simulink model "aero_guidance_targetwith315"  (R2026a)
settings: Solver=FixedStepAuto  StopTime=20  FixedStep=0.001  AbsTol=1e-6
PreLoadFcn:
  | aero_guid_dat
StopFcn:
  | aero_guid_plot
values from neighbouring files (symbols this model uses):
  d2r = pi/180    (= 0.0174532925199)    [aero_guid_plot.m]
  target_dt = 0.01    [rl_target_params.m]
undefined symbols (not defined in the file or in its folder): alpha_sch, alpha_vec, Beamwidth, Cm_alpha, Cm_el, Cm_q, Cx_alpha, Cz_alpha, Cz_el, d_ref, fin_max, fin_min, g, h_ini, K, K_r, Ka, Kg, Ki, Ks, l_acc, M_sch, Mach_vec, max_acc, max_gimbal, min_gimbal, omegaDotMax, omegaPhysMax, pos_tgt, q_ini, S_ref, Thrust, tors, v_ini, v_tgt, wgyro, wn_hom, x_ini
libraries: aerolibasang x3, simulink x2, aerolibanim x1, aerolibatmos2 x1, aerolibactuator x1, rllib x1
(part 1 of 2)
CloseFcn:
  | h=findobj('type','figure');if ~isempty(h);close(h);end
Description:
  | Dynamics of a missile engaging a target which is flying straight and level
settings Model: ExtModeTrigMode=oneshot  ExtModeArmWhenConnect=off  ExtModeAutoUpdateStatusClock=off  Creator=The MathWorks, Inc.  LastModifiedBy=신예현
settings DataIOCC: StateSaveName=xbase  OutputSaveName=ybase  SignalLoggingName=sigsOut
settings OptimizationCC: InitFltsAndDblsToZero=on
settings DebuggingCC: SaveWithParameterizedLinksMsg=none  SignalResolutionControl=TryResolveAllWithWarning  MultiTaskDSMMsg=warning  MultiTaskCondExecSysMsg=none  SigSpecEnsureSampleTimeMsg=none
settings HardwareCC: ProdHWDeviceType=32-bit Generic
settings GRTTargetCC: TargetFcnLib=ansi_tfl_tmw.mat  CombineOutputUpdateFcns=off  GRTInterface=on
settings ConfigComp: CovMetricSettings=d

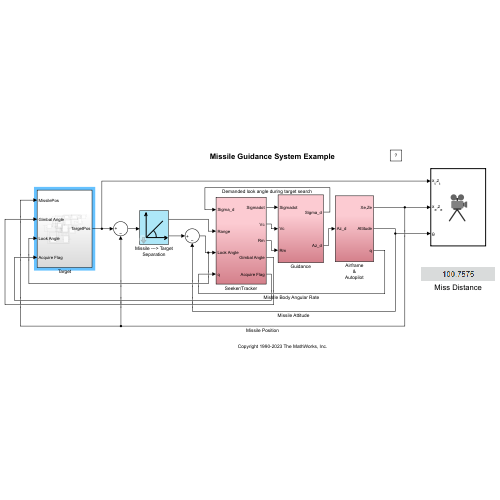
[thumbnail: Simulink's stored preview of the top-level diagram]
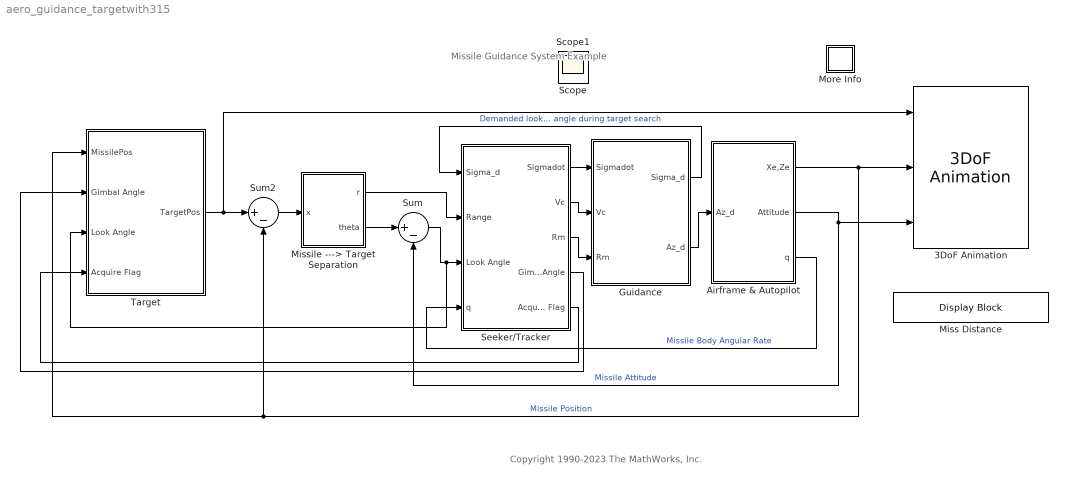
== system aero_guidance_targetwith315 ==
  note: Copyright 1990-2023 The MathWorks, Inc.
  note: Missile Guidance System Example
  3DoF Animation : aerolibanim/3DoF Animation  u1=[0 5000 -2000 2000 -5050 -3500]  u2=0.01  u3=2.0  u5=Fixed position  u6=[2500 8000 -4000]  u7=35  u8=on
  Airframe & Autopilot : Subsystem
  Guidance : Subsystem
  Miss Distance : DisplayBlock  LabelPosition=Hide  Transparency=1  GridColor=[0.0, 0.0, 0.0]
  Missile ---> Target Separation : Subsystem  mask(Cart2Polar){}
      mask help:
      | Transformation from cartesian to polar coordinates.
      | [x, y] -> [r, theta]
      |
      | r = sqrt(x^2 + y^2);
      | theta = atan(y/x);
      mask Help: Unmask this block for more help.
      mask Display: plot(0,0,100,100,[24,20,15,20,20],[85,95,85,95,20],[80,20,95,85,95,85],[70,20,20,15,20,24],[56,56,55,52,50,46],[20,26,31,35,38,42])
  More Info : Subsystem
      settings: OpenFcn=showExample('simulink_aerospace/DesigningAGuidanceSystemInMATLABAndSimulinkExample')
      mask Display: disp('?')
  Seeker/Tracker : Subsystem
  Sum : Sum  Inputs=|+-  InputSameDT=on  SaturateOnIntegerOverflow=on  OutDataTypeStr=Inherit: Same as first input
  Sum2 : Sum  Inputs=|+-  InputSameDT=on  SaturateOnIntegerOverflow=on  OutDataTypeStr=Inherit: Same as first input
  Target : Subsystem
  Scope : Scope
  Scope1 : Scope
  wires:
  Missile ---> Target Separation/2(theta) -> Sum/1
  Guidance/2(Az_d) -> Airframe & Autopilot/1(Az_d)
  Seeker/Tracker/2(Vc) -> Guidance/2(Vc)
  Seeker/Tracker/3(Rm) -> Guidance/3(Rm)
  Seeker/Tracker/1(Sigmadot) -> Guidance/1(Sigmadot)
  Sum/1 -> Target/3(Look Angle), Seeker/Tracker/3(Look Angle)
  Airframe & Autopilot/3(q) -> Seeker/Tracker/4(q)  "Missile Body Angular Rate"
  Guidance/1(Sigma_d) -> Seeker/Tracker/1(Sigma_d)  "Demanded look angle during target search"
  Missile ---> Target Separation/1(r) -> Seeker/Tracker/2(Range)
  Airframe & Autopilot/1(Xe,Ze) -> Target/1(MissilePos), Sum2/2, 3DoF Animation/2  "Missile Position"
  Airframe & Autopilot/2(Attitude) -> Sum/2, 3DoF Animation/3  "Missile Attitude"
  Sum2/1 -> Missile ---> Target Separation/1(x)
  Target/1(TargetPos) -> 3DoF Animation/1, Sum2/1
  Seeker/Tracker/4(Gimbal Angle) -> Target/2(Gimbal Angle)
  Seeker/Tracker/5(Acquire Flag) -> Target/4(Acquire Flag)

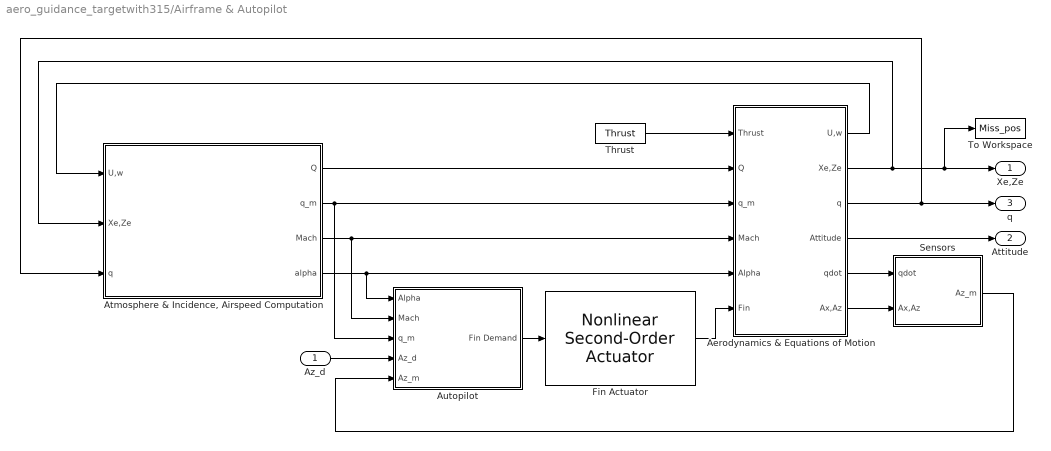
== system aero_guidance_targetwith315/Airframe & Autopilot ==
  Az_d : Inport
  Aerodynamics & Equations of Motion : Subsystem
  "Atmosphere & Incidence, Airspeed Computation" : Subsystem
  Autopilot : Subsystem
  Fin Actuator : aerolibactuator/Nonlinear Second-Order Actuator  wn_fin=wn_fin  z_fin=z_fin  fin_max=fin_max  fin_min=fin_min  fin_maxrate=fin_maxrate  fin_act_0=fin_act_0  fin_act_vel=0
  Sensors : Subsystem
  Thrust : Constant  Value=Thrust
  To Workspace : ToWorkspace  VariableName=Miss_pos  SaveFormat=Structure With Time  SampleTime=-1
  Xe,Ze : Outport  InitialOutput=0  VectorParamsAs1DForOutWhenUnconnected=off
  Attitude : Outport  Port=2  InitialOutput=0  VectorParamsAs1DForOutWhenUnconnected=off
  q : Outport  Port=3  InitialOutput=0  VectorParamsAs1DForOutWhenUnconnected=off
  wires:
  Thrust/1 -> Aerodynamics & Equations of Motion/1(Thrust)
  Aerodynamics & Equations of Motion/3(q) -> q/1, "Atmosphere & Incidence, Airspeed Computation"/3(q)
  Aerodynamics & Equations of Motion/2(Xe,Ze) -> To Workspace/1, Xe,Ze/1, "Atmosphere & Incidence, Airspeed Computation"/2(Xe,Ze)
  "Atmosphere & Incidence, Airspeed Computation"/3(Mach) -> Aerodynamics & Equations of Motion/4(Mach), Autopilot/2(Mach)
  Aerodynamics & Equations of Motion/1(U,w) -> "Atmosphere & Incidence, Airspeed Computation"/1(U,w)
  "Atmosphere & Incidence, Airspeed Computation"/1(Q) -> Aerodynamics & Equations of Motion/2(Q)
  "Atmosphere & Incidence, Airspeed Computation"/4(alpha) -> Autopilot/1(Alpha), Aerodynamics & Equations of Motion/5(Alpha)
  "Atmosphere & Incidence, Airspeed Computation"/2(q_m) -> Aerodynamics & Equations of Motion/3(q_m), Autopilot/3(q_m)
  Aerodynamics & Equations of Motion/4(Attitude) -> Attitude/1
  Aerodynamics & Equations of Motion/5(qdot) -> Sensors/1(qdot)
  Aerodynamics & Equations of Motion/6(Ax,Az) -> Sensors/2(Ax,Az)
  Autopilot/1(Fin Demand) -> Fin Actuator/1
  Fin Actuator/1 -> Aerodynamics & Equations of Motion/6(Fin)
  Az_d/1 -> Autopilot/4(Az_d)
  Sensors/1(Az_m) -> Autopilot/5(Az_m)

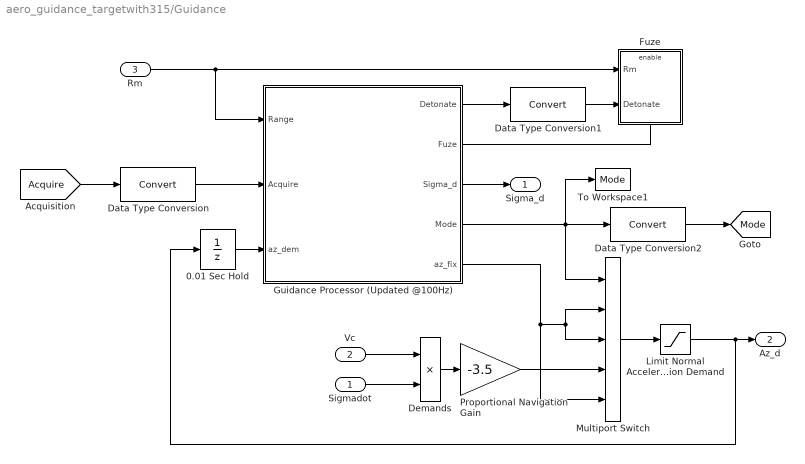
== system aero_guidance_targetwith315/Guidance ==
  Sigmadot : Inport
  Vc : Inport  Port=2
  Rm : Inport  Port=3
  0.01 Sec Hold : UnitDelay  SampleTime=0.01
  Data Type Conversion : DataTypeConversion  SaturateOnIntegerOverflow=off  RndMeth=Floor
  Data Type Conversion1 : DataTypeConversion  SaturateOnIntegerOverflow=off  RndMeth=Floor
  Data Type Conversion2 : DataTypeConversion  SaturateOnIntegerOverflow=off  RndMeth=Floor
  Demands : Product  InputSameDT=on  SaturateOnIntegerOverflow=on  OutDataTypeStr=Inherit: Same as first input
  Fuze : Subsystem  TreatAsAtomicUnit=on
  Guidance Processor (Updated @100Hz) : Stateflow chart  TreatAsAtomicUnit=on
  "Limit Normal Acceleration Demand " : Saturate  UpperLimit=max_acc  LowerLimit=-max_acc
  Multiport Switch : MultiPortSwitch  Inputs=4
  Proportional Navigation Gain : Gain  Gain=-3.5  SaturateOnIntegerOverflow=on  OutDataTypeStr=Inherit: Same as input  ParamDataTypeStr=Inherit: Same as input
  To Workspace1 : ToWorkspace  VariableName=Mode  SaveFormat=Structure With Time
  Sigma_d : Outport  VectorParamsAs1DForOutWhenUnconnected=off
  Az_d : Outport  Port=2  VectorParamsAs1DForOutWhenUnconnected=off
  tag scope: Mode=global
  wires:
  Guidance Processor (Updated @100Hz)/3(Sigma_d) -> Sigma_d/1
  [Acquire] -> Data Type Conversion/1
  Multiport Switch/1 -> "Limit Normal Acceleration Demand "/1
  Guidance Processor (Updated @100Hz)/1(Detonate) -> Data Type Conversion1/1
  "Limit Normal Acceleration Demand "/1 -> Az_d/1, 0.01 Sec Hold/1
  Guidance Processor (Updated @100Hz)/5(az_fix) -> Multiport Switch/2, Multiport Switch/3, Multiport Switch/5
  0.01 Sec Hold/1 -> Guidance Processor (Updated @100Hz)/3(az_dem)
  Sigmadot/1 -> Demands/2
  Proportional Navigation Gain/1 -> Multiport Switch/4
  Vc/1 -> Demands/1
  Demands/1 -> Proportional Navigation Gain/1
  Rm/1 -> Fuze/1(Rm), Guidance Processor (Updated @100Hz)/1(Range)
  Guidance Processor (Updated @100Hz)/2(Fuze) -> Fuze/Enable
  Guidance Processor (Updated @100Hz)/4(Mode) -> Data Type Conversion2/1, To Workspace1/1, Multiport Switch/1
  Data Type Conversion/1 -> Guidance Processor (Updated @100Hz)/2(Acquire)
  Data Type Conversion1/1 -> Fuze/2(Detonate)
  Data Type Conversion2/1 -> [Mode]

== system aero_guidance_targetwith315/Missile ---> Target Separation ==
  x : Inport
  Range : Fcn  Expr=hypot(u[1],u[2])
  Sightline Angle : Fcn  Expr=atan2(-u[2],u[1])
  r : Outport  InitialOutput=0  VectorParamsAs1DForOutWhenUnconnected=off
  theta : Outport  Port=2  InitialOutput=0  VectorParamsAs1DForOutWhenUnconnected=off
  wires:
  x/1 -> Sightline Angle/1, Range/1
  Range/1 -> r/1
  Sightline Angle/1 -> theta/1

== system aero_guidance_targetwith315/More Info ==

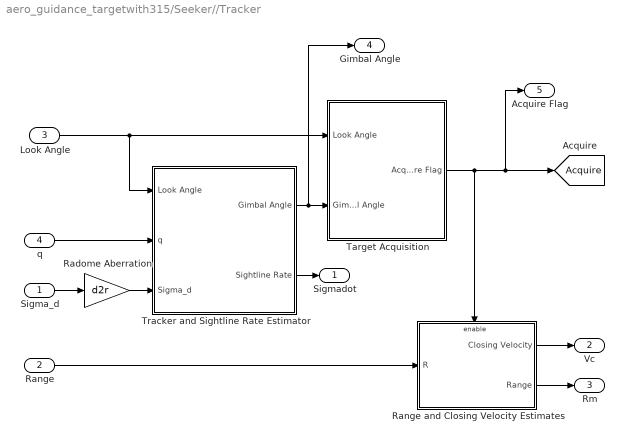
== system aero_guidance_targetwith315/Seeker//Tracker ==
  Sigma_d : Inport
  Range : Inport  Port=2
  Look Angle : Inport  Port=3
  q : Inport  Port=4
  Radome Aberration : Gain  Gain=d2r  SaturateOnIntegerOverflow=on  OutDataTypeStr=Inherit: Same as input  ParamDataTypeStr=Inherit: Same as input
  Range and Closing Velocity Estimates : Subsystem  TreatAsAtomicUnit=on
  Target Acquisition : Subsystem
  Tracker and Sightline Rate Estimator : Subsystem
  Sigmadot : Outport  VectorParamsAs1DForOutWhenUnconnected=off
  Vc : Outport  Port=2  VectorParamsAs1DForOutWhenUnconnected=off
  Rm : Outport  Port=3  VectorParamsAs1DForOutWhenUnconnected=off
  Gimbal Angle : Outport  Port=4
  Acquire Flag : Outport  Port=5
  tag scope: Acquire=global
  wires:
  Tracker and Sightline Rate Estimator/2(Sightline Rate) -> Sigmadot/1
  Radome Aberration/1 -> Tracker and Sightline Rate Estimator/3(Sigma_d)
  Tracker and Sightline Rate Estimator/1("Gimbal Angle ") -> Target Acquisition/2(Gimbal Angle), Gimbal Angle/1
  Target Acquisition/1(Acquire Flag) -> Acquire Flag/1, [Acquire], Range and Closing Velocity Estimates/Enable
  q/1 -> Tracker and Sightline Rate Estimator/2(q)
  Look Angle/1 -> Target Acquisition/1(Look Angle), Tracker and Sightline Rate Estimator/1(Look Angle)
  Range/1 -> Range and Closing Velocity Estimates/1(R)
  Range and Closing Velocity Estimates/2(Range) -> Rm/1
  Range and Closing Velocity Estimates/1(Closing Velocity) -> Vc/1
  Sigma_d/1 -> Radome Aberration/1

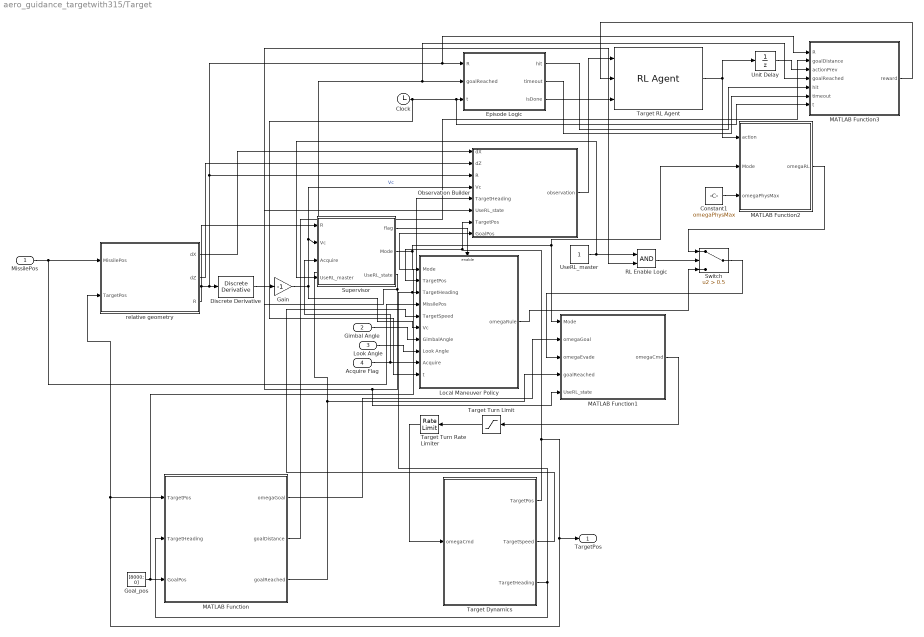
== system aero_guidance_targetwith315/Target ==
  MissilePos : Inport
  Gimbal Angle : Inport  Port=2
  Look Angle : Inport  Port=3
  Acquire Flag : Inport  Port=4
  Clock : Clock
  Constant1 : Constant  Value=omegaPhysMax
  Discrete Derivative : simulink/Discrete/Discrete Derivative  gainval=1.0  ICPrevScaledInput=0.01  OutMin=[]  OutMax=[]  OutDataType=fixdt(1, 16)  OutScaling=2^-10  DoSatur=off
  Episode Logic : MATLAB Function  TreatAsAtomicUnit=on
  Gain : Gain  Gain=-1
  Goal_pos : Constant  Value=[8000; 0]  VectorParams1D=off
  Local Maneuver Policy : Subsystem  TreatAsAtomicUnit=on
  MATLAB Function : MATLAB Function  TreatAsAtomicUnit=on
  MATLAB Function1 : MATLAB Function  TreatAsAtomicUnit=on
  MATLAB Function2 : MATLAB Function  TreatAsAtomicUnit=on
  MATLAB Function3 : MATLAB Function  TreatAsAtomicUnit=on
  Observation Builder : MATLAB Function  TreatAsAtomicUnit=on
  RL Enable Logic : Logic  AllPortsSameDT=off  OutDataTypeStr=boolean
  Supervisor : Stateflow chart  TreatAsAtomicUnit=on
  Switch : Switch  Criteria=u2 > Threshold  Threshold=0.5  SaturateOnIntegerOverflow=off  InputSameDT=off
  Target Dynamics : Subsystem
  Target RL Agent : rllib/RL Agent  Agent=agentObj  ExternalActionAsInput=off  ProvideLastAction=off  ProvideCumRwd=off  TreatAsDirectFeedthrough=on  UseStrictObservationDataTypes=off
  Target Turn Limit : Saturate  UpperLimit=omegaPhysMax  LowerLimit=-omegaPhysMax
  Target Turn Rate Limiter : RateLimiter  RisingSlewLimit=omegaDotMax  FallingSlewLimit=-omegaDotMax  SampleTimeMode=inherited
  Unit Delay : UnitDelay  SampleTime=target_dt
  UseRL_master : Constant
  relative geometry : Subsystem
  TargetPos : Outport
  wires:
  MissilePos/1 -> relative geometry/1(MissilePos), Local Maneuver Policy/4(MissilePos)
  Discrete Derivative/1 -> Gain/1
  relative geometry/3(R) -> Supervisor/1(R), Episode Logic/1(R), MATLAB Function3/1(R), Observation Builder/3(R), Discrete Derivative/1
  Gain/1 -> Observation Builder/4(Vc), Supervisor/2(Vc), Local Maneuver Policy/6(Vc)  "Vc"
  Supervisor/1(flag) -> Local Maneuver Policy/Enable
  Supervisor/2(Mode) -> Local Maneuver Policy/1(Mode), MATLAB Function2/2(Mode), MATLAB Function1/1(Mode)
  Target Dynamics/1(TargetPos) -> Observation Builder/7(TargetPos), Local Maneuver Policy/2(TargetPos), MATLAB Function/1(TargetPos), relative geometry/2(TargetPos), TargetPos/1
  relative geometry/1(dX) -> Observation Builder/1(dX)
  relative geometry/2(dZ) -> Observation Builder/2(dZ)
  Target Dynamics/3(TargetHeading) -> Observation Builder/5(TargetHeading), Local Maneuver Policy/3(TargetHeading), MATLAB Function/2(TargetHeading)
  MATLAB Function/2(goalDistance) -> MATLAB Function3/2(goalDistance)
  MATLAB Function/3(goalReached) -> MATLAB Function3/4(goalReached), Episode Logic/2(goalReached), MATLAB Function1/4(goalReached)
  Goal_pos/1 -> Observation Builder/8(GoalPos), MATLAB Function/3(GoalPos)
  MATLAB Function/1(omegaGoal) -> MATLAB Function1/2(omegaGoal)
  MATLAB Function1/1(omegaCmd) -> Target Turn Limit/1
  Target Turn Limit/1 -> Target Turn Rate Limiter/1
  Target Turn Rate Limiter/1 -> Target Dynamics/1(omegaCmd)
  Local Maneuver Policy/1(omegaRule) -> Switch/3
  Switch/1 -> MATLAB Function1/3(omegaEvade)
  UseRL_master/1 -> Supervisor/4(UseRL_master), RL Enable Logic/1
  Observation Builder/1(observation) -> Target RL Agent/1
  Target RL Agent/1 -> MATLAB Function2/1(action), Unit Delay/1
  MATLAB Function2/1(omegaRL) -> Switch/1
  Clock/1 -> MATLAB Function3/7(t), Episode Logic/3(t), Local Maneuver Policy/10(t)
  Episode Logic/3(isDone) -> Target RL Agent/3
  Unit Delay/1 -> MATLAB Function3/3(actionPrev)
  Episode Logic/1(hit) -> MATLAB Function3/5(hit)
  Episode Logic/2(timeout) -> MATLAB Function3/6(timeout)
  MATLAB Function3/1(reward) -> Target RL Agent/2
  Gimbal Angle/1 -> Local Maneuver Policy/7(GimbalAngle)
  Acquire Flag/1 -> Supervisor/3(Acquire), Local Maneuver Policy/9(Acquire)
  Constant1/1 -> MATLAB Function2/3(omegaPhysMax)
  Look Angle/1 -> Local Maneuver Policy/8(Look Angle)
  Supervisor/3(UseRL_state) -> Observation Builder/6(UseRL_state), MATLAB Function1/5(UseRL_state), RL Enable Logic/2
  RL Enable Logic/1 -> Switch/2
  Target Dynamics/2(TargetSpeed) -> Local Maneuver Policy/5(TargetSpeed)

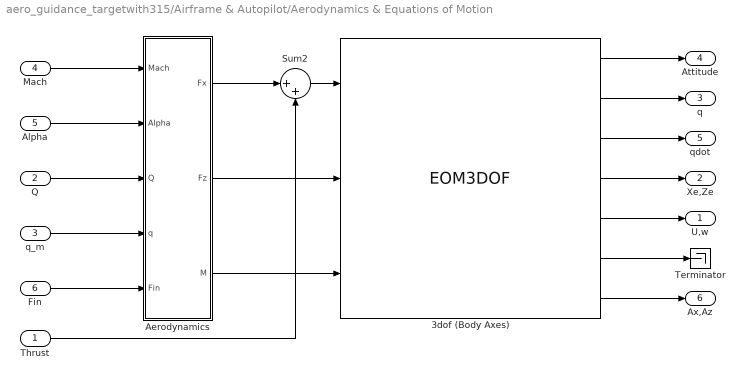
== system aero_guidance_targetwith315/Airframe & Autopilot/Aerodynamics & Equations of Motion ==
  Thrust : Inport
  Q : Inport  Port=2
  q_m : Inport  Port=3
  Mach : Inport  Port=4
  Alpha : Inport  Port=5
  Fin : Inport  Port=6
  3dof (Body Axes) : EOM3DOF  v_ini=v_ini  theta_ini=theta_ini  q_ini=q_ini  alpha_ini=alpha_ini  pos_ini=[x_ini -h_ini]  mass=mass  Iyy=Iyy  g=g  abi_flag=on
  Aerodynamics : Subsystem
  Sum2 : Sum  Inputs=|++  InputSameDT=on  SaturateOnIntegerOverflow=on  OutDataTypeStr=Inherit: Same as first input
  Terminator : Terminator
  U,w : Outport  InitialOutput=0  VectorParamsAs1DForOutWhenUnconnected=off
  Xe,Ze : Outport  Port=2  InitialOutput=0  VectorParamsAs1DForOutWhenUnconnected=off
  q : Outport  Port=3  InitialOutput=0  VectorParamsAs1DForOutWhenUnconnected=off
  Attitude : Outport  Port=4  InitialOutput=0  VectorParamsAs1DForOutWhenUnconnected=off
  qdot : Outport  Port=5  InitialOutput=0  VectorParamsAs1DForOutWhenUnconnected=off
  Ax,Az : Outport  Port=6  InitialOutput=0  VectorParamsAs1DForOutWhenUnconnected=off
  wires:
  Aerodynamics/3(" M") -> 3dof (Body Axes)/3
  Sum2/1 -> 3dof (Body Axes)/1
  Fin/1 -> Aerodynamics/5(Fin)
  Aerodynamics/2(Fz) -> 3dof (Body Axes)/2
  Aerodynamics/1(Fx) -> Sum2/1
  Thrust/1 -> Sum2/2
  q_m/1 -> Aerodynamics/4(q)
  Mach/1 -> Aerodynamics/1(Mach)
  Q/1 -> Aerodynamics/3(Q)
  Alpha/1 -> Aerodynamics/2(Alpha)
  3dof (Body Axes)/7 -> Ax,Az/1
  3dof (Body Axes)/6 -> Terminator/1
  3dof (Body Axes)/5 -> U,w/1
  3dof (Body Axes)/4 -> Xe,Ze/1
  3dof (Body Axes)/3 -> qdot/1
  3dof (Body Axes)/2 -> q/1
  3dof (Body Axes)/1 -> Attitude/1

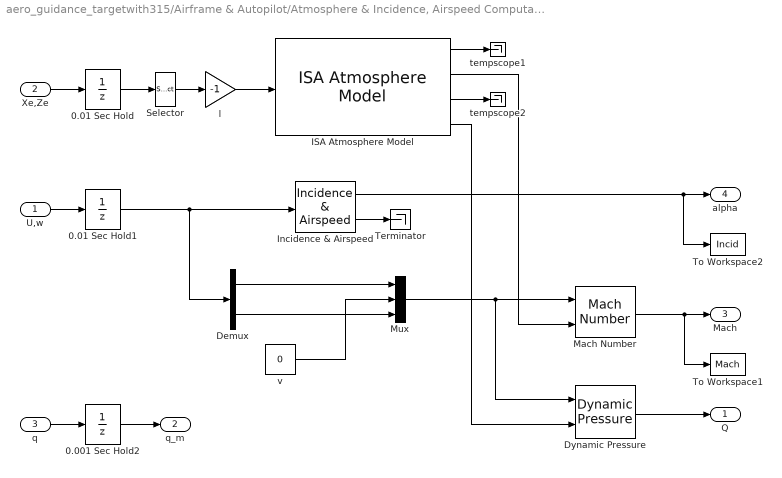
== system aero_guidance_targetwith315/Airframe & Autopilot/Atmosphere & Incidence, Airspeed Computation ==
  U,w : Inport
  Xe,Ze : Inport  Port=2
  q : Inport  Port=3
  0.001 Sec Hold2 : UnitDelay  InitialCondition=q_ini  SampleTime=0.001
  0.01 Sec Hold : UnitDelay  InitialCondition=[x_ini -h_ini]  SampleTime=0.01
  0.01 Sec Hold1 : UnitDelay  InitialCondition=[v_ini 0]  SampleTime=0.01
  Demux : Demux  Outputs=2
  Dynamic Pressure : aerolibasang/Dynamic Pressure
  ISA Atmosphere Model : aerolibatmos2/ISA Atmosphere Model  useExtended=off  action=Warning  custom=off  viscosityOut=off  g=9.80665  gamma=1.4  R=287.0531  L=0.0065  h_trop=11000  h_strat=20000  rho0=1.225  P0=101325  T0=288.15  h0=0  S=110.4  Tref=273.15  muref=1.716e-5
  Incidence & Airspeed : aerolibasang/Incidence  & Airspeed
  Mach Number : aerolibasang/Mach Number
  Mux : Mux  Inputs=3
  Selector : Selector  InputPortWidth=2  IndexOptions=Index vector (dialog)  Indices=[2]  OutputSizes=1
  Terminator : Terminator
  To Workspace1 : ToWorkspace  VariableName=Mach  SaveFormat=Structure With Time  SampleTime=-1
  To Workspace2 : ToWorkspace  VariableName=Incid  SaveFormat=Structure With Time  SampleTime=-1
  l : Gain  Gain=-1  SaturateOnIntegerOverflow=on  OutDataTypeStr=Inherit: Same as input  ParamDataTypeStr=Inherit: Same as input
  tempscope1 : Terminator
  tempscope2 : Terminator
  v : Constant  Value=0
  Q : Outport
  q_m : Outport  Port=2
  Mach : Outport  Port=3
  alpha : Outport  Port=4
  wires:
  U,w/1 -> 0.01 Sec Hold1/1
  Incidence & Airspeed/1 -> To Workspace2/1, alpha/1
  Demux/1 -> Mux/1
  Demux/2 -> Mux/3
  v/1 -> Mux/2
  Mux/1 -> Mach Number/1, Dynamic Pressure/1
  Incidence & Airspeed/2 -> Terminator/1
  ISA Atmosphere Model/4 -> Dynamic Pressure/2
  Mach Number/1 -> To Workspace1/1, Mach/1
  Dynamic Pressure/1 -> Q/1
  0.01 Sec Hold1/1 -> Incidence & Airspeed/1, Demux/1
  0.01 Sec Hold/1 -> Selector/1
  l/1 -> ISA Atmosphere Model/1
  ISA Atmosphere Model/1 -> tempscope1/1
  ISA Atmosphere Model/3 -> tempscope2/1
  Selector/1 -> l/1
  Xe,Ze/1 -> 0.01 Sec Hold/1
  ISA Atmosphere Model/2 -> Mach Number/2
  0.001 Sec Hold2/1 -> q_m/1
  q/1 -> 0.001 Sec Hold2/1

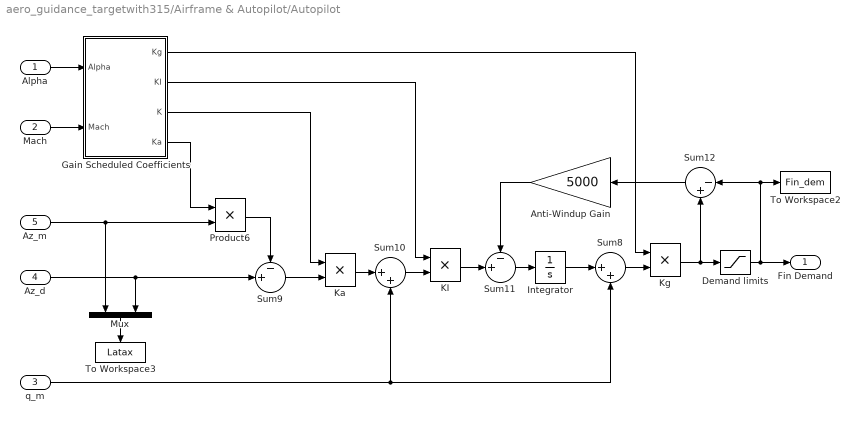
== system aero_guidance_targetwith315/Airframe & Autopilot/Autopilot ==
  Alpha : Inport
  Mach : Inport  Port=2
  q_m : Inport  Port=3
  Az_d : Inport  Port=4
  Az_m : Inport  Port=5
  Anti-Windup Gain : Gain  Gain=5000  SaturateOnIntegerOverflow=on  OutDataTypeStr=Inherit: Same as input  ParamDataTypeStr=Inherit: Same as input
  "Demand limits " : Saturate  UpperLimit=fin_max  LowerLimit=fin_min
  Gain Scheduled Coefficients : Subsystem
  Integrator : Integrator
  KI : Product  InputSameDT=on  SaturateOnIntegerOverflow=on  OutDataTypeStr=Inherit: Same as first input
  Ka : Product  InputSameDT=on  SaturateOnIntegerOverflow=on  OutDataTypeStr=Inherit: Same as first input
  Kg : Product  InputSameDT=on  SaturateOnIntegerOverflow=on  OutDataTypeStr=Inherit: Same as first input
  Mux : Mux  Inputs=2
  Product6 : Product  InputSameDT=on  SaturateOnIntegerOverflow=on  OutDataTypeStr=Inherit: Same as first input
  Sum10 : Sum  Inputs=|++  InputSameDT=on  SaturateOnIntegerOverflow=on  OutDataTypeStr=Inherit: Same as first input
  Sum11 : Sum  Inputs=-+|  InputSameDT=on  SaturateOnIntegerOverflow=on  OutDataTypeStr=Inherit: Same as first input
  Sum12 : Sum  Inputs=|-+  InputSameDT=on  SaturateOnIntegerOverflow=on  OutDataTypeStr=Inherit: Same as first input
  Sum8 : Sum  Inputs=|++  InputSameDT=on  SaturateOnIntegerOverflow=on  OutDataTypeStr=Inherit: Same as first input
  Sum9 : Sum  Inputs=-+|  InputSameDT=on  SaturateOnIntegerOverflow=on  OutDataTypeStr=Inherit: Same as first input
  To Workspace2 : ToWorkspace  VariableName=Fin_dem  SaveFormat=Structure With Time  SampleTime=-1
  To Workspace3 : ToWorkspace  VariableName=Latax  SaveFormat=Structure With Time  SampleTime=-1
  Fin Demand : Outport  InitialOutput=0  VectorParamsAs1DForOutWhenUnconnected=off
  wires:
  Mach/1 -> Gain Scheduled Coefficients/2(Mach)
  Alpha/1 -> Gain Scheduled Coefficients/1(Alpha)
  Kg/1 -> Sum12/2, "Demand limits "/1
  Gain Scheduled Coefficients/1("Kg ") -> Kg/1
  Gain Scheduled Coefficients/3("K ") -> Ka/1
  Gain Scheduled Coefficients/2("KI ") -> KI/1
  Anti-Windup Gain/1 -> Sum11/1
  Sum8/1 -> Kg/2
  Integrator/1 -> Sum8/1
  Sum11/1 -> Integrator/1
  Product6/1 -> Sum9/1
  Sum9/1 -> Ka/2
  Ka/1 -> Sum10/1
  Sum10/1 -> KI/2
  KI/1 -> Sum11/2
  Sum12/1 -> Anti-Windup Gain/1
  Az_d/1 -> Mux/2, Sum9/2
  Mux/1 -> To Workspace3/1
  q_m/1 -> Sum10/2, Sum8/2
  "Demand limits "/1 -> Fin Demand/1, Sum12/1, To Workspace2/1
  Az_m/1 -> Mux/1, Product6/2
  Gain Scheduled Coefficients/4("Ka ") -> Product6/1

== system aero_guidance_targetwith315/Airframe & Autopilot/Sensors ==
  qdot : Inport
  Ax,Az : Inport  Port=2
  Selector : Selector  InputPortWidth=2  IndexOptions=Index vector (dialog)  Indices=[2]  OutputSizes=1
  Sum : Sum  Inputs=-+|  InputSameDT=on  SaturateOnIntegerOverflow=on  OutDataTypeStr=Inherit: Same as first input
  l : Gain  Gain=l_acc  SaturateOnIntegerOverflow=on  OutDataTypeStr=Inherit: Same as input  ParamDataTypeStr=Inherit: Same as input
  Az_m : Outport  InitialOutput=0  VectorParamsAs1DForOutWhenUnconnected=off
  wires:
  Selector/1 -> Sum/2
  Ax,Az/1 -> Selector/1
  l/1 -> Sum/1
  Sum/1 -> Az_m/1  "Accelerometer"
  qdot/1 -> l/1

== system aero_guidance_targetwith315/Guidance/Fuze ==
  Rm : Inport
  Detonate : Inport  Port=2
  Enable : EnablePort
  Closest Approach : simulink/Logic and Bit Operations/Compare To Zero  relop=>=  OutDataTypeStr=boolean
  Data Type Conversion : DataTypeConversion  OutDataTypeStr=double  SaturateOnIntegerOverflow=off  RndMeth=Floor
  Derivative : Derivative
  Hit Crossing : HitCross  HitCrossingDirection=rising
  Logical Operator : Logic  Operator=OR  IconShape=distinctive  OutDataTypeStr=boolean
  Memory : Memory
  Miss distance : Subsystem  TreatAsAtomicUnit=on
  Stop Simulation : Stop
  wires:
  Derivative/1 -> Closest Approach/1
  Detonate/1 -> Logical Operator/1
  Rm/1 -> Miss distance/1(In1), Derivative/1
  Closest Approach/1 -> Logical Operator/2
  Memory/1 -> Stop Simulation/1
  Hit Crossing/1 -> Miss distance/Trigger, Memory/1
  Data Type Conversion/1 -> Hit Crossing/1
  Logical Operator/1 -> Data Type Conversion/1

== system aero_guidance_targetwith315/Seeker//Tracker/Range and Closing Velocity Estimates ==
  R : Inport
  Enable : EnablePort  StatesWhenEnabling=reset
  Bandwidth of Estimator : Gain  Gain=wn_hom  SaturateOnIntegerOverflow=on  OutDataTypeStr=Inherit: Same as input  ParamDataTypeStr=Inherit: Same as input
  Initialized at acquisition : Integrator  InitialConditionSource=external
  Rdot ---> Vc : Gain  Gain=-1  SaturateOnIntegerOverflow=on  OutDataTypeStr=Inherit: Same as input  ParamDataTypeStr=Inherit: Same as input
  Sum : Sum  Inputs=|+-  InputSameDT=on  SaturateOnIntegerOverflow=on  OutDataTypeStr=Inherit: Same as first input
  Closing Velocity : Outport  InitialOutput=0  VectorParamsAs1DForOutWhenUnconnected=off
  Range : Outport  Port=2  InitialOutput=0  VectorParamsAs1DForOutWhenUnconnected=off
  wires:
  R/1 -> Range/1, Initialized at acquisition/2, Sum/1
  Sum/1 -> Bandwidth of Estimator/1
  Initialized at acquisition/1 -> Sum/2
  Bandwidth of Estimator/1 -> Rdot ---> Vc/1, Initialized at acquisition/1
  Rdot ---> Vc/1 -> Closing Velocity/1

== system aero_guidance_targetwith315/Seeker//Tracker/Target Acquisition ==
  Look Angle : Inport
  Gimbal Angle : Inport  Port=2
  Abs : Abs
  Beamwidth : Constant  Value=Beamwidth/2
  Mux : Mux  Inputs=2
  Relational Operator : RelationalOperator  Operator=<  OutDataTypeStr=boolean
  Sum : Sum  Inputs=+-  InputSameDT=on  SaturateOnIntegerOverflow=on  OutDataTypeStr=Inherit: Same as first input
  To Workspace2 : ToWorkspace  VariableName=Gimbal  SaveFormat=Structure With Time  SampleTime=-1
  Acquire Flag : Outport  VectorParamsAs1DForOutWhenUnconnected=off
  wires:
  Look Angle/1 -> Sum/2, Mux/2
  Gimbal Angle/1 -> Sum/1, Mux/1
  Mux/1 -> To Workspace2/1
  Sum/1 -> Abs/1
  Beamwidth/1 -> Relational Operator/2
  Relational Operator/1 -> Acquire Flag/1
  Abs/1 -> Relational Operator/1

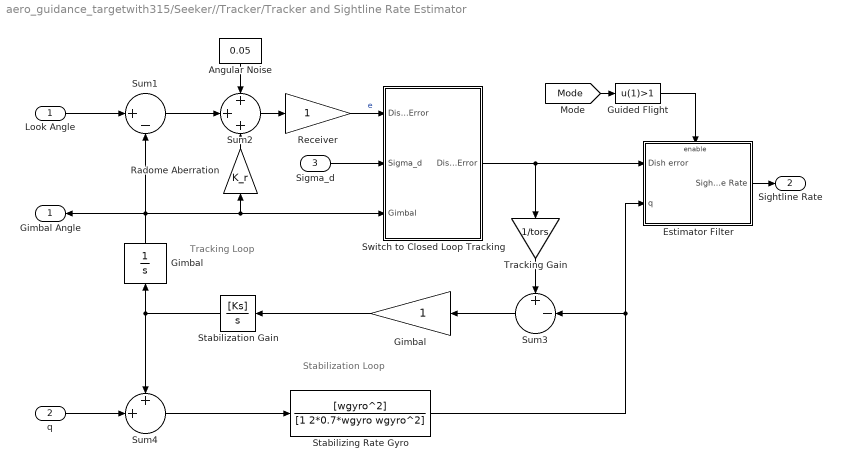
== system aero_guidance_targetwith315/Seeker//Tracker/Tracker and Sightline Rate Estimator ==
  note: Stabilization Loop
  note: Tracking Loop
  Look Angle : Inport
  q : Inport  Port=2
  Sigma_d : Inport  Port=3
  Angular Noise : Constant  Value=0.05
  Estimator Filter : Subsystem  TreatAsAtomicUnit=on
  Gimbal : Gain  SaturateOnIntegerOverflow=on  OutDataTypeStr=Inherit: Same as input  ParamDataTypeStr=Inherit: Same as input
  "Gimbal " : Integrator  LimitOutput=on  UpperSaturationLimit=max_gimbal  LowerSaturationLimit=min_gimbal
  Guided Flight : Fcn  Expr=u(1)>1
  Radome Aberration : Gain  Gain=K_r  SaturateOnIntegerOverflow=on  OutDataTypeStr=Inherit: Same as input  ParamDataTypeStr=Inherit: Same as input
  Receiver : Gain  SaturateOnIntegerOverflow=on  OutDataTypeStr=Inherit: Same as input  ParamDataTypeStr=Inherit: Same as input
  Stabilization Gain : TransferFcn  Numerator=[Ks]  Denominator=[1 0]
  Stabilizing Rate Gyro : TransferFcn  Numerator=[wgyro^2]  Denominator=[1 2*0.7*wgyro wgyro^2]
  Sum1 : Sum  Inputs=|+-  InputSameDT=on  SaturateOnIntegerOverflow=on  OutDataTypeStr=Inherit: Same as first input
  Sum2 : Sum  Inputs=+++  InputSameDT=on  SaturateOnIntegerOverflow=on  OutDataTypeStr=Inherit: Same as first input
  Sum3 : Sum  Inputs=+-|  InputSameDT=on  SaturateOnIntegerOverflow=on  OutDataTypeStr=Inherit: Same as first input
  Sum4 : Sum  Inputs=++|  InputSameDT=on  SaturateOnIntegerOverflow=on  OutDataTypeStr=Inherit: Same as first input
  Switch to Closed Loop Tracking : Subsystem
  Tracking Gain : Gain  Gain=1/tors  SaturateOnIntegerOverflow=on  OutDataTypeStr=Inherit: Same as input  ParamDataTypeStr=Inherit: Same as input
  "Gimbal Angle " : Outport  VectorParamsAs1DForOutWhenUnconnected=off
  Sightline Rate : Outport  Port=2  VectorParamsAs1DForOutWhenUnconnected=off
  wires:
  "Gimbal "/1 -> Sum1/2, Radome Aberration/1, Switch to Closed Loop Tracking/3(Gimbal), "Gimbal Angle "/1
  Stabilization Gain/1 -> "Gimbal "/1, Sum4/1
  Gimbal/1 -> Stabilization Gain/1
  Look Angle/1 -> Sum1/1
  Sum2/1 -> Receiver/1
  Receiver/1 -> Switch to Closed Loop Tracking/1(Dish Error)  "e"
  Sigma_d/1 -> Switch to Closed Loop Tracking/2(Sigma_d)
  Estimator Filter/1(Sightline Rate) -> Sightline Rate/1
  Radome Aberration/1 -> Sum2/3
  Sum1/1 -> Sum2/2
  Angular Noise/1 -> Sum2/1
  Sum4/1 -> Stabilizing Rate Gyro/1
  q/1 -> Sum4/2
  Stabilizing Rate Gyro/1 -> Sum3/2, Estimator Filter/2(q)
  Sum3/1 -> Gimbal/1
  Tracking Gain/1 -> Sum3/1
  Switch to Closed Loop Tracking/1("Dish Error ") -> Tracking Gain/1, Estimator Filter/1(Dish error)
  Guided Flight/1 -> Estimator Filter/Enable
  [Mode] -> Guided Flight/1

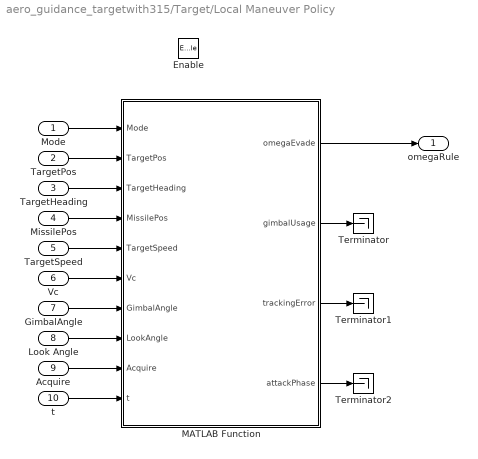
== system aero_guidance_targetwith315/Target/Local Maneuver Policy ==
  Mode : Inport
  TargetPos : Inport  Port=2
  TargetHeading : Inport  Port=3
  MissilePos : Inport  Port=4
  TargetSpeed : Inport  Port=5
  Vc : Inport  Port=6
  GimbalAngle : Inport  Port=7
  Look Angle : Inport  Port=8
  Acquire : Inport  Port=9
  t : Inport  Port=10
  Enable : EnablePort  StatesWhenEnabling=reset
  MATLAB Function : MATLAB Function  TreatAsAtomicUnit=on
  Terminator : Terminator
  Terminator1 : Terminator
  Terminator2 : Terminator
  omegaRule : Outport  OutputWhenDisabled=reset  InitialOutput=0
  wires:
  Mode/1 -> MATLAB Function/1(Mode)
  MATLAB Function/1(omegaEvade) -> omegaRule/1
  TargetPos/1 -> MATLAB Function/2(TargetPos)
  TargetHeading/1 -> MATLAB Function/3(TargetHeading)
  MissilePos/1 -> MATLAB Function/4(MissilePos)
  Vc/1 -> MATLAB Function/6(Vc)
  GimbalAngle/1 -> MATLAB Function/7(GimbalAngle)
  Acquire/1 -> MATLAB Function/9(Acquire)
  t/1 -> MATLAB Function/10(t)
  MATLAB Function/2(gimbalUsage) -> Terminator/1
  MATLAB Function/3(trackingError) -> Terminator1/1
  MATLAB Function/4(attackPhase) -> Terminator2/1
  Look Angle/1 -> MATLAB Function/8(LookAngle)
  TargetSpeed/1 -> MATLAB Function/5(TargetSpeed)

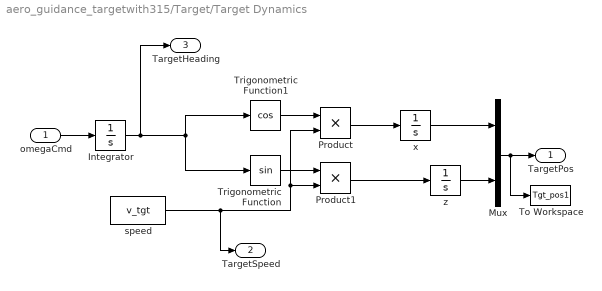
== system aero_guidance_targetwith315/Target/Target Dynamics ==
  omegaCmd : Inport
  Integrator : Integrator
  Mux : Mux  Inputs=2
  Product : Product  InputSameDT=on  SaturateOnIntegerOverflow=on  OutDataTypeStr=Inherit: Same as first input
  Product1 : Product  InputSameDT=on  SaturateOnIntegerOverflow=on  OutDataTypeStr=Inherit: Same as first input
  To Workspace : ToWorkspace  VariableName=Tgt_pos1  SaveFormat=Structure  SampleTime=-1
  Trigonometric Function : Trigonometry
  Trigonometric Function1 : Trigonometry  Operator=cos
  speed : Constant  Value=v_tgt
  x : Integrator  InitialCondition=pos_tgt(1)
  z : Integrator  InitialCondition=pos_tgt(2)
  TargetPos : Outport
  TargetSpeed : Outport  Port=2
  TargetHeading : Outport  Port=3
  wires:
  omegaCmd/1 -> Integrator/1
  Integrator/1 -> Trigonometric Function/1, Trigonometric Function1/1, TargetHeading/1
  x/1 -> Mux/1
  z/1 -> Mux/2
  Trigonometric Function/1 -> Product1/1
  speed/1 -> TargetSpeed/1, Product/2, Product1/2
  Product1/1 -> z/1
  Product/1 -> x/1
  Trigonometric Function1/1 -> Product/1
  Mux/1 -> TargetPos/1, To Workspace/1

== system aero_guidance_targetwith315/Target/relative geometry ==
  MissilePos : Inport
  TargetPos : Inport  Port=2
  MATLAB Function : MATLAB Function  TreatAsAtomicUnit=on
  dX : Outport
  dZ : Outport  Port=2
  R : Outport  Port=3
  wires:
  MissilePos/1 -> MATLAB Function/1(MissilePos)
  TargetPos/1 -> MATLAB Function/2(TargetPos)
  MATLAB Function/1(dX) -> dX/1
  MATLAB Function/2(dZ) -> dZ/1
  MATLAB Function/3(R) -> R/1

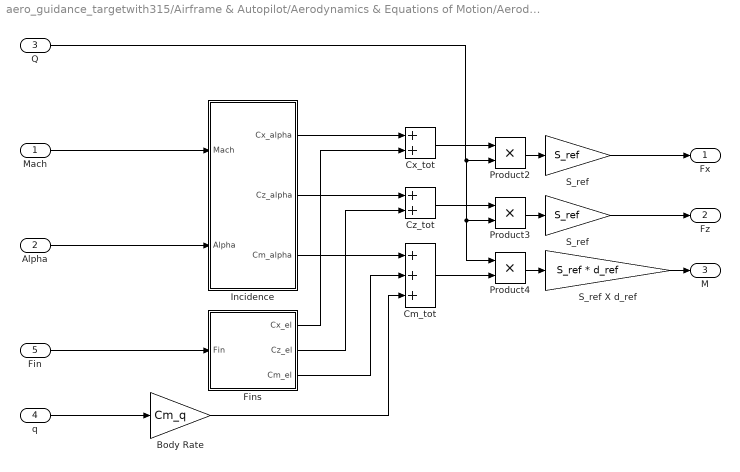
== system aero_guidance_targetwith315/Airframe & Autopilot/Aerodynamics & Equations of Motion/Aerodynamics ==
  Mach : Inport
  Alpha : Inport  Port=2
  Q : Inport  Port=3
  q : Inport  Port=4
  Fin : Inport  Port=5
  Body Rate : Gain  Gain=Cm_q  SaturateOnIntegerOverflow=on  OutDataTypeStr=Inherit: Same as input  ParamDataTypeStr=Inherit: Same as input
  Cm_tot : Sum  Inputs=+++  InputSameDT=on  SaturateOnIntegerOverflow=on  OutDataTypeStr=Inherit: Same as first input
  Cx_tot : Sum  InputSameDT=on  SaturateOnIntegerOverflow=on  OutDataTypeStr=Inherit: Same as first input
  Cz_tot : Sum  InputSameDT=on  SaturateOnIntegerOverflow=on  OutDataTypeStr=Inherit: Same as first input
  Fins : Subsystem
  Incidence : Subsystem
  Product2 : Product  InputSameDT=on  SaturateOnIntegerOverflow=on  OutDataTypeStr=Inherit: Same as first input
  Product3 : Product  InputSameDT=on  SaturateOnIntegerOverflow=on  OutDataTypeStr=Inherit: Same as first input
  Product4 : Product  InputSameDT=on  SaturateOnIntegerOverflow=on  OutDataTypeStr=Inherit: Same as first input
  S_ref : Gain  Gain=S_ref  SaturateOnIntegerOverflow=on  OutDataTypeStr=Inherit: Same as input  ParamDataTypeStr=Inherit: Same as input
  "S_ref " : Gain  Gain=S_ref  SaturateOnIntegerOverflow=on  OutDataTypeStr=Inherit: Same as input  ParamDataTypeStr=Inherit: Same as input
  S_ref X d_ref : Gain  Gain=S_ref * d_ref  SaturateOnIntegerOverflow=on  OutDataTypeStr=Inherit: Same as input  ParamDataTypeStr=Inherit: Same as input
  Fx : Outport  InitialOutput=[0]  VectorParamsAs1DForOutWhenUnconnected=off
  Fz : Outport  Port=2  InitialOutput=0  VectorParamsAs1DForOutWhenUnconnected=off
  " M" : Outport  Port=3  InitialOutput=0  VectorParamsAs1DForOutWhenUnconnected=off
  wires:
  Incidence/1(Cx_alpha) -> Cx_tot/1
  Fins/1(Cx_el) -> Cx_tot/2
  Incidence/2(Cz_alpha) -> Cz_tot/1
  Fins/2(Cz_el) -> Cz_tot/2
  Incidence/3(Cm_alpha) -> Cm_tot/1
  Fins/3(Cm_el) -> Cm_tot/2
  Body Rate/1 -> Cm_tot/3
  Alpha/1 -> Incidence/2(Alpha)
  Cx_tot/1 -> Product2/1
  Cz_tot/1 -> Product3/1
  Product2/1 -> S_ref/1
  S_ref/1 -> Fx/1
  Product3/1 -> "S_ref "/1
  "S_ref "/1 -> Fz/1
  Fin/1 -> Fins/1(Fin)
  S_ref X d_ref/1 -> " M"/1
  Product4/1 -> S_ref X d_ref/1
  Cm_tot/1 -> Product4/2
  Mach/1 -> Incidence/1(Mach)
  q/1 -> Body Rate/1
  Q/1 -> Product4/1, Product3/2, Product2/2

== system aero_guidance_targetwith315/Airframe & Autopilot/Autopilot/Gain Scheduled Coefficients ==
  Alpha : Inport
  Mach : Inport  Port=2
  2-D Lookup Table : Lookup_n-D  BreakpointsForDimension1=M_sch  BreakpointsForDimension2=alpha_sch  Table=Ka  InternalRulePriority=Speed  RndMeth=Simplest
      settings: InputPortMap=u0,u1
  2-D Lookup Table1 : Lookup_n-D  BreakpointsForDimension1=M_sch  BreakpointsForDimension2=alpha_sch  Table=K  InternalRulePriority=Speed  RndMeth=Simplest
      settings: InputPortMap=u0,u1
  2-D Lookup Table2 : Lookup_n-D  BreakpointsForDimension1=M_sch  BreakpointsForDimension2=alpha_sch  Table=Ki  InternalRulePriority=Speed  RndMeth=Simplest
      settings: InputPortMap=u0,u1
  2-D Lookup Table3 : Lookup_n-D  BreakpointsForDimension1=M_sch  BreakpointsForDimension2=alpha_sch  Table=Kg  InternalRulePriority=Speed  RndMeth=Simplest
      settings: InputPortMap=u0,u1
  Abs : Abs
  "Kg " : Outport  InitialOutput=0  VectorParamsAs1DForOutWhenUnconnected=off
  "KI " : Outport  Port=2  InitialOutput=0  VectorParamsAs1DForOutWhenUnconnected=off
  "K " : Outport  Port=3  InitialOutput=0  VectorParamsAs1DForOutWhenUnconnected=off
  "Ka " : Outport  Port=4  InitialOutput=0  VectorParamsAs1DForOutWhenUnconnected=off
  wires:
  Alpha/1 -> Abs/1
  2-D Lookup Table/1 -> "Ka "/1
  2-D Lookup Table1/1 -> "K "/1
  2-D Lookup Table2/1 -> "KI "/1
  2-D Lookup Table3/1 -> "Kg "/1
  Mach/1 -> 2-D Lookup Table3/1, 2-D Lookup Table2/1, 2-D Lookup Table1/1, 2-D Lookup Table/1
  Abs/1 -> 2-D Lookup Table3/2, 2-D Lookup Table2/2, 2-D Lookup Table/2, 2-D Lookup Table1/2

== system aero_guidance_targetwith315/Guidance/Fuze/Miss distance ==
  In1 : Inport
  Trigger : TriggerPort  VariantControl=(inherit)
  Display : Display
  wires:
  In1/1 -> Display/1  "Miss Distance"

== system aero_guidance_targetwith315/Seeker//Tracker/Tracker and Sightline Rate Estimator/Estimator Filter ==
  Dish error : Inport
  q : Inport  Port=2
  Enable : EnablePort  StatesWhenEnabling=reset
  Integrator : Integrator  InitialConditionSource=external
  Sum : Sum  Inputs=|+-  InputSameDT=on  SaturateOnIntegerOverflow=on  OutDataTypeStr=Inherit: Same as first input
  Sum1 : Sum  Inputs=|+-  InputSameDT=on  SaturateOnIntegerOverflow=on  OutDataTypeStr=Inherit: Same as first input
  Sum5 : Sum  Inputs=|++  InputSameDT=on  SaturateOnIntegerOverflow=on  OutDataTypeStr=Inherit: Same as first input
  q_filt : Integrator
  wn_hom : Gain  Gain=wn_hom  SaturateOnIntegerOverflow=on  OutDataTypeStr=Inherit: Same as input  ParamDataTypeStr=Inherit: Same as input
  "wn_hom  " : Gain  Gain=wn_hom  SaturateOnIntegerOverflow=on  OutDataTypeStr=Inherit: Same as input  ParamDataTypeStr=Inherit: Same as input
  Sightline Rate : Outport  InitialOutput=0  VectorParamsAs1DForOutWhenUnconnected=off
  wires:
  Dish error/1 -> Sum/1, Integrator/2
  Sum/1 -> wn_hom/1
  Integrator/1 -> Sum/2
  Sum5/1 -> Sightline Rate/1
  wn_hom/1 -> Integrator/1, Sum5/1
  q/1 -> Sum1/1
  Sum1/1 -> "wn_hom  "/1
  "wn_hom  "/1 -> q_filt/1
  q_filt/1 -> Sum5/2, Sum1/2

== system aero_guidance_targetwith315/Seeker//Tracker/Tracker and Sightline Rate Estimator/Switch to Closed Loop Tracking ==
  Dish Error : Inport
  Sigma_d : Inport  Port=2
  Gimbal : Inport  Port=3
  Guided Flight : Fcn  Expr=u(1)>1
  Sum5 : Sum  Inputs=-+  InputSameDT=on  SaturateOnIntegerOverflow=on  OutDataTypeStr=Inherit: Same as first input
  Switch2 : Switch  Threshold=0.5
  "Dish Error " : Outport  VectorParamsAs1DForOutWhenUnconnected=off
  wires:
  [Mode] -> Guided Flight/1
  Guided Flight/1 -> Switch2/2
  Sum5/1 -> Switch2/3
  Dish Error/1 -> Switch2/1
  Switch2/1 -> "Dish Error "/1
  Sigma_d/1 -> Sum5/2
  Gimbal/1 -> Sum5/1

== system aero_guidance_targetwith315/Airframe & Autopilot/Aerodynamics & Equations of Motion/Aerodynamics/Fins ==
  Fin : Inport
  Cm : Gain  Gain=Cm_el  SaturateOnIntegerOverflow=on  OutDataTypeStr=Inherit: Same as input  ParamDataTypeStr=Inherit: Same as input
  Cx : Gain  Gain=0  SaturateOnIntegerOverflow=on  OutDataTypeStr=Inherit: Same as input  ParamDataTypeStr=Inherit: Same as input
  Cz : Gain  Gain=Cz_el  SaturateOnIntegerOverflow=on  OutDataTypeStr=Inherit: Same as input  ParamDataTypeStr=Inherit: Same as input
  Cx_el : Outport  InitialOutput=0  VectorParamsAs1DForOutWhenUnconnected=off
  Cz_el : Outport  Port=2  InitialOutput=0  VectorParamsAs1DForOutWhenUnconnected=off
  Cm_el : Outport  Port=3  InitialOutput=0  VectorParamsAs1DForOutWhenUnconnected=off
  wires:
  Fin/1 -> Cx/1, Cm/1, Cz/1
  Cx/1 -> Cx_el/1
  Cm/1 -> Cm_el/1
  Cz/1 -> Cz_el/1

== system aero_guidance_targetwith315/Airframe & Autopilot/Aerodynamics & Equations of Motion/Aerodynamics/Incidence ==
  Mach : Inport
  Alpha : Inport  Port=2
  2-D Lookup Table : Lookup_n-D  BreakpointsForDimension1=alpha_vec  BreakpointsForDimension2=Mach_vec  Table=Cx_alpha  InternalRulePriority=Speed  RndMeth=Simplest
      settings: InputPortMap=u0,u1
  2-D Lookup Table1 : Lookup_n-D  BreakpointsForDimension1=alpha_vec  BreakpointsForDimension2=Mach_vec  Table=Cz_alpha  InternalRulePriority=Speed  RndMeth=Simplest
      settings: InputPortMap=u0,u1
  2-D Lookup Table2 : Lookup_n-D  BreakpointsForDimension1=alpha_vec  BreakpointsForDimension2=Mach_vec  Table=Cm_alpha  InternalRulePriority=Speed  RndMeth=Simplest
      settings: InputPortMap=u0,u1
  Cx_alpha : Outport  InitialOutput=0  VectorParamsAs1DForOutWhenUnconnected=off
  Cz_alpha : Outport  Port=2  InitialOutput=0  VectorParamsAs1DForOutWhenUnconnected=off
  Cm_alpha : Outport  Port=3  InitialOutput=0  VectorParamsAs1DForOutWhenUnconnected=off
  wires:
  Alpha/1 -> 2-D Lookup Table/1, 2-D Lookup Table2/1, 2-D Lookup Table1/1
  2-D Lookup Table/1 -> Cx_alpha/1
  2-D Lookup Table1/1 -> Cz_alpha/1
  Mach/1 -> 2-D Lookup Table2/2, 2-D Lookup Table1/2, 2-D Lookup Table/2
  2-D Lookup Table2/1 -> Cm_alpha/1

== matlab function aero_guidance_targetwith315/Target/relative geometry/MATLAB Function ==
  data: MissilePos input; dX output; TargetPos input; dZ output; R output
function [dX, dZ, R ] = ...
    calculateGeometry(MissilePos, TargetPos)
%#codegen

% Missile position
Xm = MissilePos(1);
Zm = MissilePos(2);

% Target position
Xt = TargetPos(1);
Zt = TargetPos(2);

% Relative position: Target - Missile
dX = Xt - Xm;
dZ = Zt - Zm;

% Relative range
R = sqrt(dX^2 + dZ^2);

end

== stateflow chart aero_guidance_targetwith315/Target/Supervisor ==
  state Target_Evasion
    state Nomal_Flight
      en: Mode=0;flag=0;UseRL_state = false;
    state Threat_Confirm
      en:Mode=1;flag=0;UseRL_state = false;
    state Recovery
      en: Mode=4;flag=0;UseRL_state = false;
    state Evasive_Maneuver
      en:Mode=2;flag=1;UseRL_state = false;
    state RL_Local_Evasion
      en:Mode = 2;flag = 1;UseRL_state = true;
    state Terminal_Evasion
      en:Mode=3;flag=1;UseRL_state = false;
    (default) -> Nomal_Flight
    Recovery -> Nomal_Flight [order 1] : [after(0.5,sec) && R > 3800]
    Threat_Confirm -> Nomal_Flight [order 2] : [R >= 3000 || Vc <= 0]
    Nomal_Flight -> Threat_Confirm : [R < 3000 && Vc > 0]
    Recovery -> Threat_Confirm [order 2] : [R < 3000 && Vc > 0]
    Threat_Confirm -> Evasive_Maneuver [order 1] : [after(0.05,sec) && R < 3000 && Vc > 0]
    Evasive_Maneuver -> Recovery [order 2] : [after(1.0,sec) && R > 3800]
    Evasive_Maneuver -> Terminal_Evasion [order 1] : [R <= 1200 && Vc > 0 && R/Vc < 1.5]
    RL_Local_Evasion -> Evasive_Maneuver [order 2] : [R >= 2600 || ~UseRL_master || Acquire == 0]
    Evasive_Maneuver -> RL_Local_Evasion [order 3] : [after(0.1,sec) && UseRL_master && R < 3500 && R > 1500 && Vc > 0 && Acquire == 1]
    Terminal_Evasion -> Recovery : [after(0.8,sec) && Acquire == 1 && R > 1800]
    RL_Local_Evasion -> Terminal_Evasion [order 1] : [R <= 900 && Vc > 0 && R/Vc < 1.2]
  data: flag output; R input; Vc input size=1; Acquire input; UseRL_master input size=1; Mode output; UseRL_state output size=1 =false
